simulink model "my_pv_system_2_sc_user_interface"  (Simulink 8.4)
settings: Solver=ode3  SolverMode=SingleTasking  StartTime=0.0  StopTime=inf  FixedStep=5e-05  RelTol=1e-3
libraries: opal_lib x3, simulink x2
Description:
  | Model of a simple control system for use iin training.
settings Model: Creator=Paul Baracos  LastModifiedBy=jiang  BufferReuse=off
settings DataIOCC: SaveOutput=off  SaveTime=off  SignalLoggingName=sigsOut
settings OptimizationCC: BlockReduction=off  BooleanDataType=off  OptimizeBlockIOStorage=off  BufferReuse=off  GlobalBufferReuse=off  ExpressionFolding=off  ExpressionDepthLimit=128  LocalBlockOutputs=off  InitFltsAndDblsToZero=on
settings DebuggingCC: SaveWithParameterizedLinksMsg=none  SignalResolutionControl=TryResolveAllWithWarning  SolverPrmCheckMsg=none  MultiTaskDSMMsg=warning  MultiTaskCondExecSysMsg=none  StateNameClashWarn=none
settings HardwareCC: TargetHWDeviceType=32-bit Generic  TargetUnknown=on  ProdEqTarget=off
settings RTWCC: GenCodeOnly=on  IncludeERTFirstTime=on
settings GRTTargetCC: TargetFcnLib=ansi_tfl_tmw.mat
settings ConfigurationSet: Description=SimMechanics 2G

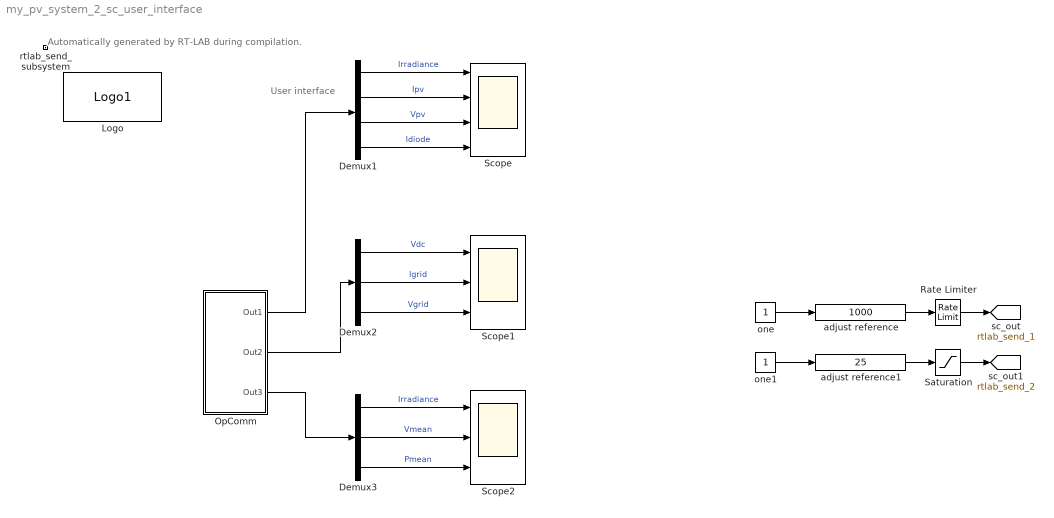
== system my_pv_system_2_sc_user_interface ==
  note: User interface
  note: Automatically generated by RT-LAB during compilation.
  Demux1 : Demux
  Demux2 : Demux  Outputs=3
  Demux3 : Demux  Outputs=3
  Logo : opal_lib/Logo1  vide=[]
  OpComm : Subsystem
      mask init:
      | opmaskdisplay('maskdisplay_block',gcb,'disp(''OpComm'')');
      mask Display:
      | patch([0 0.5 0.7 0],[1 1 0 0],[0.7 0.75 0.9]);
      | patch([1 0.53 0.73 1],[1 1 0 0],[1 0.8 0.7]);
      | plot([0 0 1 1 0],[0 1 1 0 0]);
      | disp('OpComm')
  Rate Limiter : RateLimiter  RisingSlewLimit=8000  FallingSlewLimit=-8000  SampleTimeMode=inherited  InitialCondition=1000
  Saturation : Saturate  UpperLimit=55  LowerLimit=5
  Scope : Scope  NumInputPorts=4
      settings: YMin=0~-5~-5~-5  YMax=100~5~5~5
  Scope1 : Scope  NumInputPorts=3
      settings: YMin=0~-5~-5  YMax=100~5~5
  Scope2 : Scope  NumInputPorts=3
      settings: YMin=0~-5~-5  YMax=100~5~5  SaveName=ScopeData2
  adjust reference : simulink/Math Operations/Slider Gain  low=0  gain=1000  high=1000
  adjust reference1 : simulink/Math Operations/Slider Gain  low=0  gain=25  high=60
  one : Constant
  one1 : Constant
  rtlab_send_subsystem : Subsystem  Priority=-100
      mask Display: text(0,0,'');
  tag scope: rtlab_send_1=global, rtlab_send_2=global
  wires:
  OpComm/3(Out3) -> Demux3/1
  Demux3/2 -> Scope2/2  "Vmean"
  Demux3/3 -> Scope2/3  "Pmean"
  Demux3/1 -> Scope2/1  "Irradiance"
  Demux2/1 -> Scope1/1  "Vdc"
  Demux2/3 -> Scope1/3  "Vgrid"
  Demux2/2 -> Scope1/2  "Igrid"
  Demux1/1 -> Scope/1  "Irradiance"
  Demux1/4 -> Scope/4  "Idiode"
  Demux1/3 -> Scope/3  "Vpv"
  Demux1/2 -> Scope/2  "Ipv"
  OpComm/1(Out1) -> Demux1/1
  OpComm/2(Out2) -> Demux2/1
  adjust reference1/1 -> Saturation/1
  adjust reference/1 -> Rate Limiter/1
  Saturation/1 -> [rtlab_send_2]
  Rate Limiter/1 -> [rtlab_send_1]
  one1/1 -> adjust reference1/1
  one/1 -> adjust reference/1

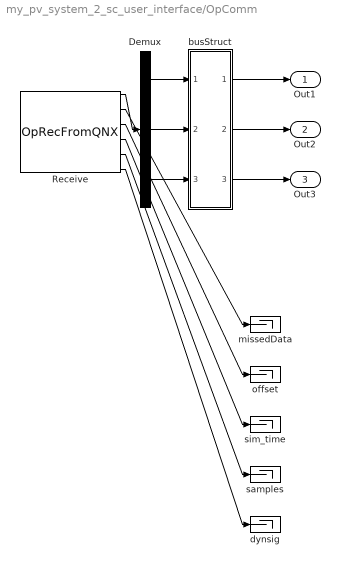
== system my_pv_system_2_sc_user_interface/OpComm ==
  Demux : Demux  Outputs="[4  3  3]"
  Receive : opal_lib/Communication/OpRecFromQNX  Node_num=1  Acqu_Group=1  Data_Width=10  Synchronization=on  Interpolation=on  Threshold=1.0  modelname=my_pv_system.mdl  sampletime=5e-05
  busStruct : Subsystem
  dynsig : Terminator
  missedData : Terminator
  offset : Terminator
  samples : Terminator
  sim_time : Terminator
  Out1 : Outport
  Out2 : Outport  Port=2
  Out3 : Outport  Port=3
  wires:
  Demux/3 -> busStruct/3(In3)
  Demux/2 -> busStruct/2(In2)
  Demux/1 -> busStruct/1(In1)
  busStruct/3(Out3) -> Out3/1
  busStruct/2(Out2) -> Out2/1
  busStruct/1(Out1) -> Out1/1
  Receive/1 -> Demux/1
  Receive/6 -> dynsig/1
  Receive/5 -> samples/1
  Receive/4 -> sim_time/1
  Receive/3 -> offset/1
  Receive/2 -> missedData/1

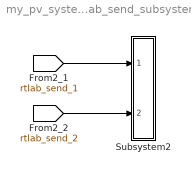
== system my_pv_system_2_sc_user_interface/rtlab_send_subsystem ==
  Subsystem2 : Subsystem
  wires:
  [rtlab_send_1] -> Subsystem2/1(In1)
  [rtlab_send_2] -> Subsystem2/2(In2)

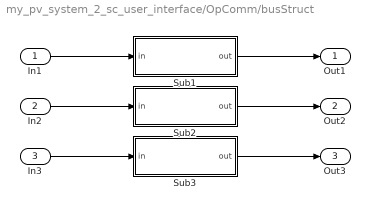
== system my_pv_system_2_sc_user_interface/OpComm/busStruct ==
  In1 : Inport
  In2 : Inport  Port=2
  In3 : Inport  Port=3
  Sub1 : Subsystem
  Sub2 : Subsystem
  Sub3 : Subsystem
  Out1 : Outport
  Out2 : Outport  Port=2
  Out3 : Outport  Port=3
  wires:
  Sub3/1(out) -> Out3/1
  In3/1 -> Sub3/1(in)
  Sub2/1(out) -> Out2/1
  In2/1 -> Sub2/1(in)
  Sub1/1(out) -> Out1/1
  In1/1 -> Sub1/1(in)

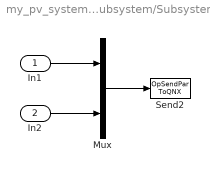
== system my_pv_system_2_sc_user_interface/rtlab_send_subsystem/Subsystem2 ==
  In1 : Inport  PortDimensions=1
  In2 : Inport  Port=2  PortDimensions=1
  Mux : Mux  Inputs=2
  Send2 : opal_lib/Communication/OpSendPar ToQNX  Node_num=1  modelname=my_pv_system
  wires:
  Mux/1 -> Send2/1
  In1/1 -> Mux/1
  In2/1 -> Mux/2

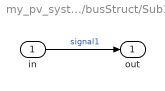
== system my_pv_system_2_sc_user_interface/OpComm/busStruct/Sub1 ==
  in : Inport
  out : Outport
  wires:
  in/1 -> out/1  "signal1"

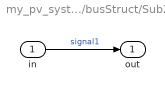
== system my_pv_system_2_sc_user_interface/OpComm/busStruct/Sub2 ==
  in : Inport
  out : Outport
  wires:
  in/1 -> out/1  "signal1"

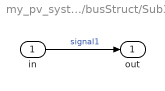
== system my_pv_system_2_sc_user_interface/OpComm/busStruct/Sub3 ==
  in : Inport
  out : Outport
  wires:
  in/1 -> out/1  "signal1"
